simulink model "EX001_FCHEV"  (R2020b)
settings: Solver=ode23tb  StartTime=0.0  StopTime=20e3  MaxStep=1  RelTol=1e-4
libraries: component_lib x75, pid_lib x3, simulink x2, base_lib x1
settings Model: Creator=maxjo65  LastModifiedBy=CJ

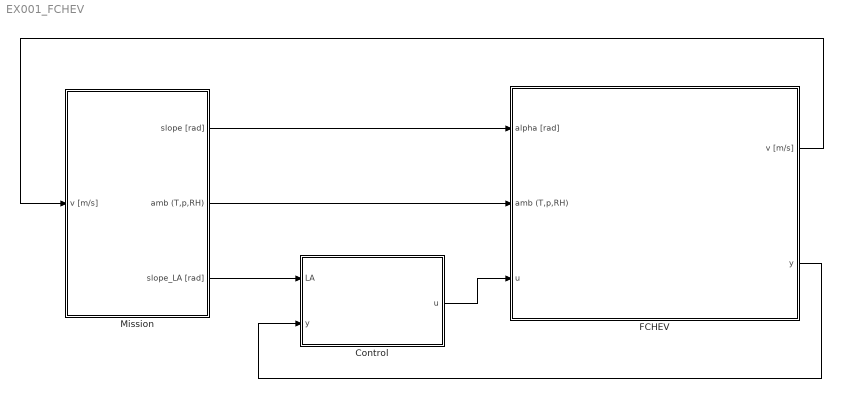
== system EX001_FCHEV ==
  Control : Subsystem
  FCHEV : Subsystem
  Mission : Subsystem
  wires:
  FCHEV/1(v [m/s]) -> Mission/1(v [m/s])
  Mission/1(slope [rad]) -> FCHEV/1(alpha [rad])
  Mission/2(amb (T,p,RH)) -> FCHEV/2(amb (T,p,RH))
  Mission/3(slope_LA [rad]) -> Control/1(LA)
  Control/1(u) -> FCHEV/3(u)
  FCHEV/2(y) -> Control/2(y)

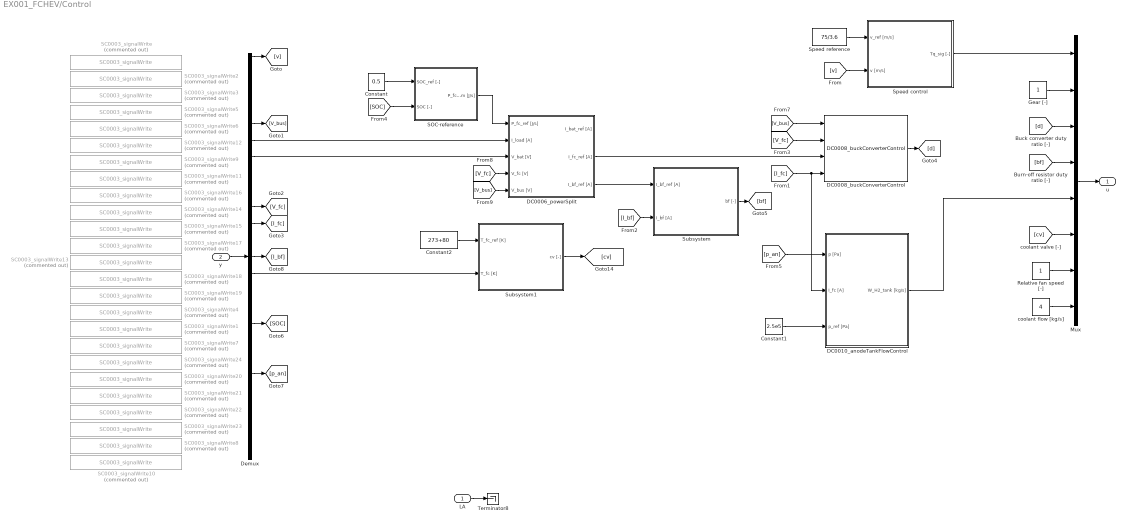
== system EX001_FCHEV/Control ==
  LA : Inport
  y : Inport  Port=2
  Constant : Constant  Value=0.5
  Constant1 : Constant  Value=2.5e5
  Constant2 : Constant  Value=273+80
  DC0006_powerSplit : Subsystem  mask{P_fc_max=400e3, P_fc_min=10e3, T_s=1, I_bt_max=600, I_bt_min=-300}
      mask prompts: P_fc_max "Max. FC power [J/s]:"; P_fc_min "Min. FC power [J/s]:"; T_s "FC Dynamic load time constant [s]:"; I_bt_max "Max. battery current [A]:"; I_bt_min "Min. battery current [A]:"
  DC0008_buckConverterControl : component_lib/Data & Control/DC0008_buckConverterControl  SystemSampleTime=-1  VariantActivationTime=update diagram  Latency=0  AutoFrameSizeCalculation=off
  DC0010_anodeTankFlowControl : Subsystem  mask{n_cell=450*2}
      mask prompts: n_cell "Nr. of cells [-]"
  Demux : Demux  Outputs=25
  Gear [-] : Constant
  Mux : Mux  Inputs=8
  Relative fan speed [-] : Constant
  SC0003_signalWrite : component_lib/Data & Control/SC0003_signalWrite  Commented=on  SigName=velocity
  SC0003_signalWrite1 : component_lib/Data & Control/SC0003_signalWrite  Commented=on  SigName=stateOfCharge
  SC0003_signalWrite10 : component_lib/Data & Control/SC0003_signalWrite  Commented=on  SigName=empty
  SC0003_signalWrite11 : component_lib/Data & Control/SC0003_signalWrite  Commented=on  SigName=batteryCurrent
  SC0003_signalWrite12 : component_lib/Data & Control/SC0003_signalWrite  Commented=on  SigName=loadCurrent
  SC0003_signalWrite13 : component_lib/Data & Control/SC0003_signalWrite  Commented=on  SigName=burnOffCurrent
  SC0003_signalWrite14 : component_lib/Data & Control/SC0003_signalWrite  Commented=on  SigName=fuelCellVoltage
  SC0003_signalWrite15 : component_lib/Data & Control/SC0003_signalWrite  Commented=on  SigName=fuelCellCurrent
  SC0003_signalWrite16 : component_lib/Data & Control/SC0003_signalWrite  Commented=on  SigName=batteryPower
  SC0003_signalWrite17 : component_lib/Data & Control/SC0003_signalWrite  Commented=on  SigName=fuelCellPower
  SC0003_signalWrite18 : component_lib/Data & Control/SC0003_signalWrite  Commented=on  SigName=fuelCellTemperature
  SC0003_signalWrite19 : component_lib/Data & Control/SC0003_signalWrite  Commented=on  SigName=motorTemperature
  SC0003_signalWrite2 : component_lib/Data & Control/SC0003_signalWrite  Commented=on  SigName=motorTorque
  SC0003_signalWrite20 : component_lib/Data & Control/SC0003_signalWrite  Commented=on  SigName=anodeSupplyPressure
  SC0003_signalWrite21 : component_lib/Data & Control/SC0003_signalWrite  Commented=on  SigName=anodeSupplyHumidity
  SC0003_signalWrite22 : component_lib/Data & Control/SC0003_signalWrite  Commented=on  SigName=cathodePressure
  SC0003_signalWrite23 : component_lib/Data & Control/SC0003_signalWrite  Commented=on  SigName=cathodeHumidity
  SC0003_signalWrite24 : component_lib/Data & Control/SC0003_signalWrite  Commented=on  SigName=anodePrimaryFlow
  SC0003_signalWrite3 : component_lib/Data & Control/SC0003_signalWrite  Commented=on  SigName=maxMotorTorque
  SC0003_signalWrite4 : component_lib/Data & Control/SC0003_signalWrite  Commented=on  SigName=powerElectronicsTemperature
  SC0003_signalWrite5 : component_lib/Data & Control/SC0003_signalWrite  Commented=on  SigName=motorSpeed
  SC0003_signalWrite6 : component_lib/Data & Control/SC0003_signalWrite  Commented=on  SigName=busVoltage
  SC0003_signalWrite7 : component_lib/Data & Control/SC0003_signalWrite  Commented=on  SigName=anodePrimaryPressure
  SC0003_signalWrite8 : component_lib/Data & Control/SC0003_signalWrite  Commented=on  SigName=anodePrimaryPressure
  SC0003_signalWrite9 : component_lib/Data & Control/SC0003_signalWrite  Commented=on  SigName=batteryVoltage
  SOC-reference : Subsystem
  Speed control : Subsystem
  Speed reference : Constant  Value=75/3.6
  Subsystem : Subsystem
  Subsystem1 : Subsystem
  Terminator8 : Terminator
  coolant flow [kg/s] : Constant  Value=4
  u : Outport
  wires:
  y/1 -> Demux/1
  Demux/1 -> [v]
  Mux/1 -> u/1
  Speed reference/1 -> Speed control/1(v_ref [m/s])
  Speed control/1(Tq_sig [-]) -> Mux/1
  [v] -> Speed control/2(v [m/s])
  Gear [-]/1 -> Mux/2
  [V_bus] -> DC0008_buckConverterControl/1
  [V_fc] -> DC0008_buckConverterControl/2
  DC0006_powerSplit/2(I_fc_ref [A]) -> DC0008_buckConverterControl/3
  DC0006_powerSplit/3(I_bf_ref [A]) -> Subsystem/1(I_bf_ref [A])
  Demux/6 -> DC0006_powerSplit/2(I_load [A])
  Demux/7 -> DC0006_powerSplit/3(V_bat [V])
  Demux/5 -> [V_bus]
  Demux/10 -> [V_fc]
  Demux/11 -> [I_fc]
  DC0008_buckConverterControl/1 -> [d]
  [d] -> Mux/3
  [bf] -> Mux/4
  Subsystem/1(bf [-]) -> [bf]
  [cv] -> Mux/6
  [I_fc] -> DC0010_anodeTankFlowControl/2(I_fc [A]), DC0008_buckConverterControl/4
  [I_bf] -> Subsystem/2(I_bf [A])
  Constant2/1 -> Subsystem1/1(T_fc_ref [K])
  Subsystem1/1(cv [-]) -> [cv]
  Demux/13 -> [I_bf]
  Demux/14 -> Subsystem1/2(T_fc [K])
  Relative fan speed [-]/1 -> Mux/7
  coolant flow [kg/s]/1 -> Mux/8
  LA/1 -> Terminator8/1
  [V_fc] -> DC0006_powerSplit/4(V_fc [V])
  [V_bus] -> DC0006_powerSplit/5(V_bus [V])
  Demux/17 -> [SOC]
  SOC-reference/1(P_fc_nom [J/s]) -> DC0006_powerSplit/1(P_fc_ref [J/s])
  Constant/1 -> SOC-reference/1(SOC_ref [-])
  [SOC] -> SOC-reference/2(SOC [-])
  DC0010_anodeTankFlowControl/1(W_H2_tank [kg/s]) -> Mux/5
  Demux/20 -> [p_an]
  [p_an] -> DC0010_anodeTankFlowControl/1(p [Pa])
  Constant1/1 -> DC0010_anodeTankFlowControl/3(p_ref [Pa])

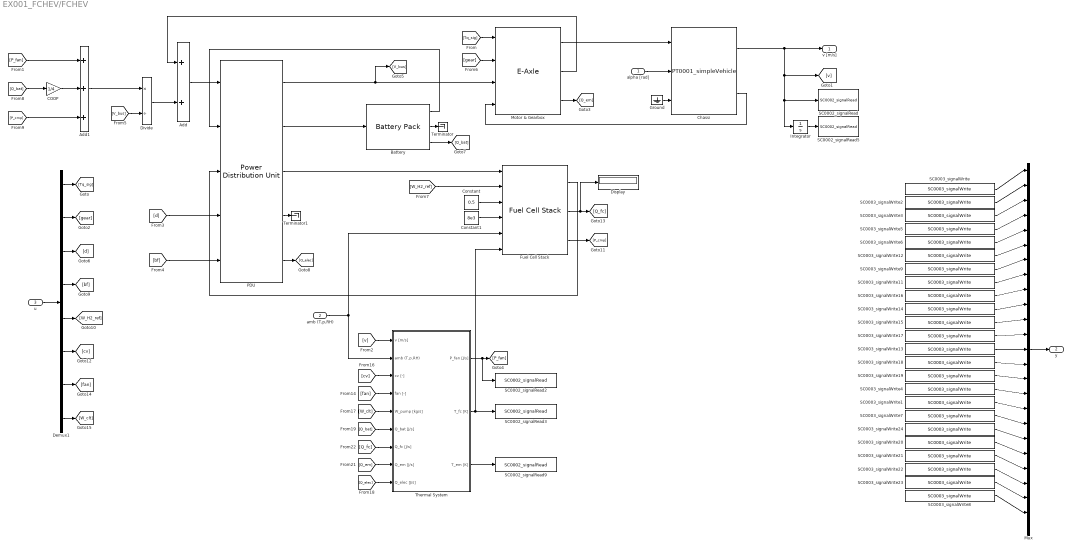
== system EX001_FCHEV/FCHEV ==
  alpha [rad] : Inport
  amb (T,p,RH) : Inport  Port=2
  u : Inport  Port=3
  Add : Sum
  Add1 : Sum  Inputs=3
  Battery : component_lib/Battery Pack  SOC_0=0.5  Nx=80  Ny=100  T_bat=273 + 20
  COOP : Gain  Gain=1/4
  Chassi : component_lib/Powertrain/PT0001_simpleVehicle  m=40e3  r_w=0.5  A_f=10  C_d=0.5  rho_air=1.225  c_r0=0.0060  c_r1=2.3e-7  gain=600  v0=75/3.6  x0=0
  Constant : Constant  Value=0.5
  Constant1 : Constant  Value=8e3
  Demux1 : Demux  Outputs=8
  Display : Display
  Divide : Product  Inputs=*/
  Fuel Cell Stack : component_lib/Fuel Cell Stack  n=450*2
  Ground : Ground
  Integrator : Integrator
  Motor & Gearbox : component_lib/E-Axle  n=3
  Mux : Mux  Inputs=25
  PDU : component_lib/Power Distribution Unit  R_bf=0.5
  SC0002_signalRead : component_lib/Data & Control/SC0002_signalRead  SigName=velocity
  SC0002_signalRead2 : component_lib/Data & Control/SC0002_signalRead  SigName=fanPower
  SC0002_signalRead3 : component_lib/Data & Control/SC0002_signalRead  SigName=fuelCellTemperature
  SC0002_signalRead5 : component_lib/Data & Control/SC0002_signalRead  SigName=distance
  SC0002_signalRead9 : component_lib/Data & Control/SC0002_signalRead  SigName=motorTemperature
  SC0003_signalWrite : component_lib/Data & Control/SC0003_signalWrite  SigName=velocity
  SC0003_signalWrite1 : component_lib/Data & Control/SC0003_signalWrite  SigName=stateOfCharge
  SC0003_signalWrite11 : component_lib/Data & Control/SC0003_signalWrite  SigName=batteryCurrent
  SC0003_signalWrite12 : component_lib/Data & Control/SC0003_signalWrite  SigName=loadCurrent
  SC0003_signalWrite13 : component_lib/Data & Control/SC0003_signalWrite  SigName=burnOffCurrent
  SC0003_signalWrite14 : component_lib/Data & Control/SC0003_signalWrite  SigName=fuelCellVoltage
  SC0003_signalWrite15 : component_lib/Data & Control/SC0003_signalWrite  SigName=fuelCellCurrent
  SC0003_signalWrite16 : component_lib/Data & Control/SC0003_signalWrite  SigName=batteryPower
  SC0003_signalWrite17 : component_lib/Data & Control/SC0003_signalWrite  SigName=fuelCellPower
  SC0003_signalWrite18 : component_lib/Data & Control/SC0003_signalWrite  SigName=fuelCellTemperature
  SC0003_signalWrite19 : component_lib/Data & Control/SC0003_signalWrite  SigName=motorTemperature
  SC0003_signalWrite2 : component_lib/Data & Control/SC0003_signalWrite  SigName=motorTorque
  SC0003_signalWrite20 : component_lib/Data & Control/SC0003_signalWrite  SigName=anodeSupplyPressure
  SC0003_signalWrite21 : component_lib/Data & Control/SC0003_signalWrite  SigName=anodeSupplyHumidity
  SC0003_signalWrite22 : component_lib/Data & Control/SC0003_signalWrite  SigName=cathodePressure
  SC0003_signalWrite23 : component_lib/Data & Control/SC0003_signalWrite  SigName=cathodeHumidity
  SC0003_signalWrite24 : component_lib/Data & Control/SC0003_signalWrite  SigName=anodePrimaryFlow
  SC0003_signalWrite3 : component_lib/Data & Control/SC0003_signalWrite  SigName=maxMotorTorque
  SC0003_signalWrite4 : component_lib/Data & Control/SC0003_signalWrite  SigName=powerElectronicsTemperature
  SC0003_signalWrite5 : component_lib/Data & Control/SC0003_signalWrite  SigName=motorSpeed
  SC0003_signalWrite6 : component_lib/Data & Control/SC0003_signalWrite  SigName=busVoltage
  SC0003_signalWrite7 : component_lib/Data & Control/SC0003_signalWrite  SigName=anodePrimaryPressure
  SC0003_signalWrite8 : component_lib/Data & Control/SC0003_signalWrite  SigName=anodePrimaryPressure
  SC0003_signalWrite9 : component_lib/Data & Control/SC0003_signalWrite  SigName=batteryVoltage
  Terminator : Terminator
  Terminator1 : Terminator
  Thermal System : Subsystem
  v [m/s] : Outport
  y : Outport  Port=2
  wires:
  Battery/1 -> PDU/2
  Fuel Cell Stack/1 -> PDU/3
  PDU/2 -> Battery/1
  PDU/3 -> Fuel Cell Stack/1
  Motor & Gearbox/3 -> [Q_em]
  Motor & Gearbox/1 -> Chassi/1
  Chassi/1 -> v [m/s]/1, [v], SC0002_signalRead/1, Integrator/1
  Chassi/2 -> Motor & Gearbox/4
  Motor & Gearbox/2 -> Add/1
  PDU/5 -> [Q_elec]
  Battery/3 -> [Q_bat]
  PDU/1 -> [V_bus], Motor & Gearbox/3
  alpha [rad]/1 -> Chassi/2
  u/1 -> Demux1/1
  Demux1/2 -> [gear]
  Demux1/1 -> [Tq_sig]
  [Tq_sig] -> Motor & Gearbox/1
  [gear] -> Motor & Gearbox/2
  Demux1/3 -> [d]
  Demux1/4 -> [bf]
  [d] -> PDU/4
  [bf] -> PDU/5
  Demux1/6 -> [cv]
  Mux/1 -> y/1
  Thermal System/2(T_fc [K]) -> Fuel Cell Stack/6, SC0002_signalRead3/1
  Demux1/7 -> [fan]
  Demux1/8 -> [W_clt]
  amb (T,p,RH)/1 -> Fuel Cell Stack/5, Thermal System/2(amb (T,p,RH))
  Thermal System/3(T_em [K]) -> SC0002_signalRead9/1
  [v] -> Thermal System/1(v [m/s])
  [fan] -> Thermal System/4(fan [-])
  [W_clt] -> Thermal System/5(W_pump [kg/s])
  [cv] -> Thermal System/3(cv [-])
  [Q_elec] -> Thermal System/9(Q_elec [J/s])
  [Q_bat] -> Thermal System/6(Q_bat [J/s])
  [Q_em] -> Thermal System/8(Q_em [J/s])
  [Q_fc] -> Thermal System/7(Q_fc [J/s])
  SC0003_signalWrite4/1 -> Mux/16
  SC0003_signalWrite2/1 -> Mux/2
  SC0003_signalWrite19/1 -> Mux/15
  SC0003_signalWrite/1 -> Mux/1
  SC0003_signalWrite17/1 -> Mux/12
  SC0003_signalWrite16/1 -> Mux/9
  SC0003_signalWrite13/1 -> Mux/13
  SC0003_signalWrite6/1 -> Mux/5
  SC0003_signalWrite15/1 -> Mux/11
  SC0003_signalWrite5/1 -> Mux/4
  SC0003_signalWrite9/1 -> Mux/7
  SC0003_signalWrite3/1 -> Mux/3
  SC0003_signalWrite11/1 -> Mux/8
  SC0003_signalWrite12/1 -> Mux/6
  SC0003_signalWrite18/1 -> Mux/14
  SC0003_signalWrite14/1 -> Mux/10
  Integrator/1 -> SC0002_signalRead5/1
  Ground/1 -> Chassi/3
  SC0003_signalWrite1/1 -> Mux/17
  Add/1 -> PDU/1
  Battery/2 -> Terminator/1
  Thermal System/1(P_fan [J/s]) -> SC0002_signalRead2/1, [P_fan]
  [Q_bat] -> COOP/1
  [P_fan] -> Add1/1
  COOP/1 -> Add1/2
  Add1/1 -> Divide/1
  Divide/1 -> Add/2
  [V_bus] -> Divide/2
  [P_cmp] -> Add1/3
  PDU/4 -> Terminator1/1
  Fuel Cell Stack/2 -> Display/1, [Q_fc]
  Fuel Cell Stack/3 -> [P_cmp]
  Constant/1 -> Fuel Cell Stack/3
  Constant1/1 -> Fuel Cell Stack/4
  Demux1/5 -> [W_H2_ref]
  [W_H2_ref] -> Fuel Cell Stack/2
  SC0003_signalWrite7/1 -> Mux/18
  SC0003_signalWrite22/1 -> Mux/22
  SC0003_signalWrite23/1 -> Mux/23
  SC0003_signalWrite21/1 -> Mux/21
  SC0003_signalWrite20/1 -> Mux/20
  SC0003_signalWrite24/1 -> Mux/19
  SC0003_signalWrite8/1 -> Mux/24

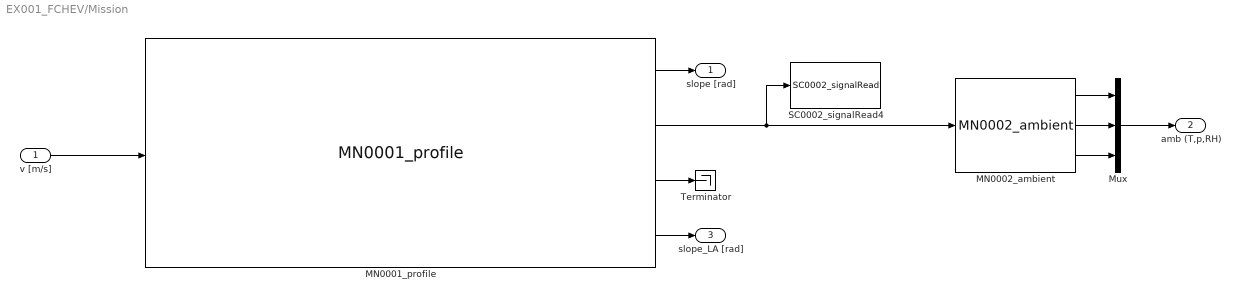
== system EX001_FCHEV/Mission ==
  v [m/s] : Inport
  MN0001_profile : component_lib/Mission/MN0001_profile  profile=KoblenzTrier.mat  x0=0  N_lookahead=100
  MN0002_ambient : component_lib/Mission/MN0002_ambient  p_0=1.01e5  T_0=273 + 45  RH_0=0.2
  Mux : Mux  Inputs=3
  SC0002_signalRead4 : component_lib/Data & Control/SC0002_signalRead  SigName=altitude
  Terminator : Terminator
  slope [rad] : Outport
  amb (T,p,RH) : Outport  Port=2
  slope_LA [rad] : Outport  Port=3
  wires:
  Mux/1 -> amb (T,p,RH)/1
  MN0001_profile/2 -> MN0002_ambient/1, SC0002_signalRead4/1
  MN0001_profile/1 -> slope [rad]/1
  MN0002_ambient/3 -> Mux/3
  MN0002_ambient/1 -> Mux/1
  MN0002_ambient/2 -> Mux/2
  v [m/s]/1 -> MN0001_profile/1
  MN0001_profile/4 -> slope_LA [rad]/1
  MN0001_profile/3 -> Terminator/1

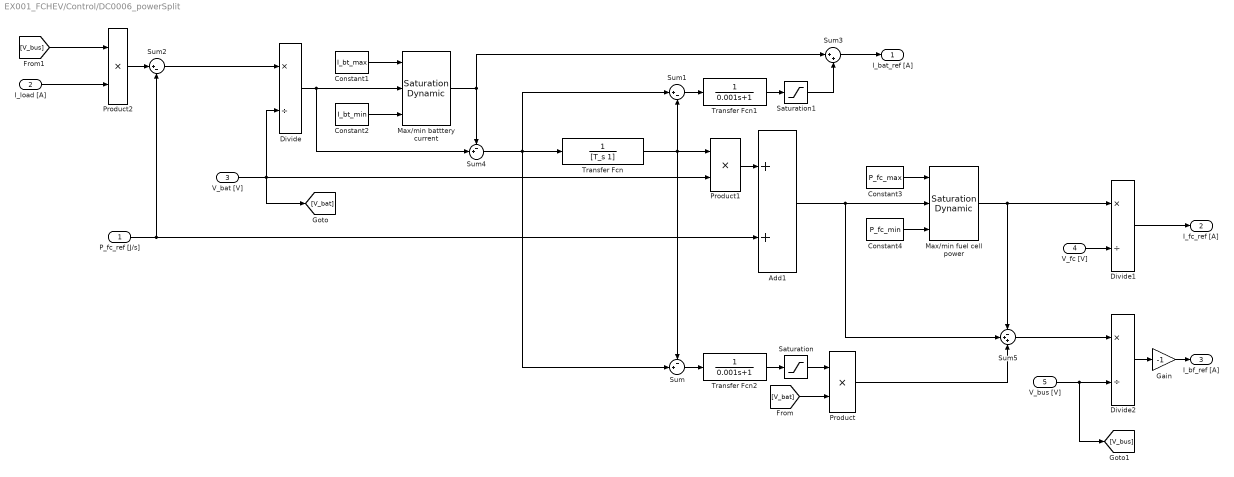
== system EX001_FCHEV/Control/DC0006_powerSplit ==
  P_fc_ref [J/s] : Inport
  I_load [A] : Inport  Port=2
  V_bat [V] : Inport  Port=3
  V_fc [V] : Inport  Port=4
  V_bus [V] : Inport  Port=5
  Add1 : Sum
  Constant1 : Constant  Value=I_bt_max
  Constant2 : Constant  Value=I_bt_min
  Constant3 : Constant  Value=P_fc_max
  Constant4 : Constant  Value=P_fc_min
  Divide : Product  Inputs=*/
  Divide1 : Product  Inputs=*/
  Divide2 : Product  Inputs=*/
  Gain : Gain  Gain=-1
  Max/min batttery current : simulink/Discontinuities/Saturation Dynamic  OutMin=[]  OutMax=[]  OutDataTypeStr=Inherit: Same as second input  OutDataType=fixdt(1, 16)  OutScaling=2^-10  DoSatur=off
  Max/min fuel cell power : simulink/Discontinuities/Saturation Dynamic  OutMin=[]  OutMax=[]  OutDataTypeStr=Inherit: Same as second input  OutDataType=fixdt(1, 16)  OutScaling=2^-10  DoSatur=off
  Product : Product
  Product1 : Product
  Product2 : Product
  Saturation : Saturate  UpperLimit=0  LowerLimit=-inf
  Saturation1 : Saturate  UpperLimit=inf  LowerLimit=0
  Sum : Sum  Inputs=-+|
  Sum1 : Sum  Inputs=|+-
  Sum2 : Sum  Inputs=|+-
  Sum3 : Sum  Inputs=|++
  Sum4 : Sum  Inputs=-+|
  Sum5 : Sum  Inputs=-++
  Transfer Fcn : TransferFcn  Denominator=[T_s 1]
  Transfer Fcn1 : TransferFcn  Denominator=[0.001 1]
  Transfer Fcn2 : TransferFcn  Denominator=[0.001 1]
  I_bat_ref [A] : Outport
  I_fc_ref [A] : Outport  Port=2
  I_bf_ref [A] : Outport  Port=3
  wires:
  Gain/1 -> I_bf_ref [A]/1
  [V_bus] -> Product2/1
  I_load [A]/1 -> Product2/2
  Product2/1 -> Sum2/1
  Transfer Fcn2/1 -> Saturation/1
  Sum/1 -> Transfer Fcn2/1
  Transfer Fcn1/1 -> Saturation1/1
  Sum1/1 -> Transfer Fcn1/1
  Sum3/1 -> I_bat_ref [A]/1
  Saturation1/1 -> Sum3/2
  Product/1 -> Sum5/3
  Saturation/1 -> Product/1
  [V_bat] -> Product/2
  Transfer Fcn/1 -> Sum/1, Product1/1, Sum1/2
  Sum4/1 -> Transfer Fcn/1, Sum/2, Sum1/1
  Max/min batttery current/1 -> Sum4/1, Sum3/1
  Product1/1 -> Add1/1
  V_fc [V]/1 -> Divide1/2
  Divide2/1 -> Gain/1
  V_bus [V]/1 -> Divide2/2, [V_bus]
  Sum5/1 -> Divide2/1
  Max/min fuel cell power/1 -> Divide1/1, Sum5/1
  Constant4/1 -> Max/min fuel cell power/3
  Constant3/1 -> Max/min fuel cell power/1
  Add1/1 -> Max/min fuel cell power/2, Sum5/2
  Constant2/1 -> Max/min batttery current/3
  Constant1/1 -> Max/min batttery current/1
  Divide/1 -> Sum4/2, Max/min batttery current/2
  P_fc_ref [J/s]/1 -> Add1/2, Sum2/2
  V_bat [V]/1 -> Divide/2, [V_bat], Product1/2
  Divide1/1 -> I_fc_ref [A]/1
  Sum2/1 -> Divide/1

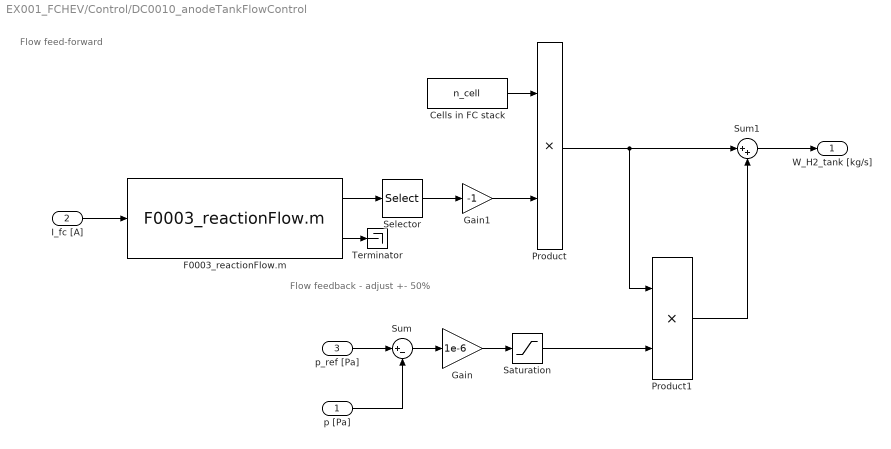
== system EX001_FCHEV/Control/DC0010_anodeTankFlowControl ==
  note: Flow feed-forward
  note: Flow feedback - adjust +- 50%
  p [Pa] : Inport
  I_fc [A] : Inport  Port=2
  p_ref [Pa] : Inport  Port=3
  Cells in FC stack : Constant  Value=n_cell
  F0003_reactionFlow.m : base_lib/F0003_pukrushpan2004/F0003_reactionFlow.m  SystemSampleTime=-1  VariantActivationTime=update diagram  Latency=0  AutoFrameSizeCalculation=off
  Gain : Gain  Gain=1e-6
  Gain1 : Gain  Gain=-1
  Product : Product
  Product1 : Product
  Saturation : Saturate
  Selector : Selector  InputPortWidth=4  IndexOptions=Index vector (dialog)  Indices=1  OutputSizes=1
  Sum : Sum  Inputs=|+-
  Sum1 : Sum  Inputs=|++
  Terminator : Terminator
  W_H2_tank [kg/s] : Outport
  wires:
  Saturation/1 -> Product1/2
  Gain/1 -> Saturation/1
  Product1/1 -> Sum1/2
  Sum/1 -> Gain/1
  Sum1/1 -> W_H2_tank [kg/s]/1
  Product/1 -> Product1/1, Sum1/1
  p [Pa]/1 -> Sum/2
  p_ref [Pa]/1 -> Sum/1
  Cells in FC stack/1 -> Product/1
  F0003_reactionFlow.m/2 -> Terminator/1
  I_fc [A]/1 -> F0003_reactionFlow.m/1
  F0003_reactionFlow.m/1 -> Selector/1
  Selector/1 -> Gain1/1
  Gain1/1 -> Product/2

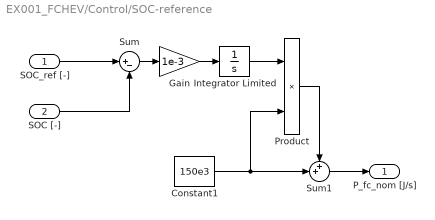
== system EX001_FCHEV/Control/SOC-reference ==
  SOC_ref [-] : Inport
  SOC [-] : Inport  Port=2
  Constant1 : Constant  Value=150e3
  Gain : Gain  Gain=1e-3
  Integrator Limited : Integrator  LimitOutput=on  UpperSaturationLimit=0.3  LowerSaturationLimit=-0.3
  Product : Product
  Sum : Sum  Inputs=|+-
  Sum1 : Sum  Inputs=++|
  P_fc_nom [J/s] : Outport
  wires:
  Product/1 -> Sum1/1
  Integrator Limited/1 -> Product/1
  Sum1/1 -> P_fc_nom [J/s]/1
  Constant1/1 -> Sum1/2, Product/2
  Sum/1 -> Gain/1
  SOC [-]/1 -> Sum/2
  Gain/1 -> Integrator Limited/1
  SOC_ref [-]/1 -> Sum/1

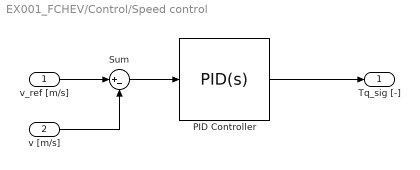
== system EX001_FCHEV/Control/Speed control ==
  v_ref [m/s] : Inport
  v [m/s] : Inport  Port=2
  PID Controller : pid_lib/PID Controller  Controller=PID  Form=Parallel  TimeDomain=Continuous-time  UseExternalTs=off  SampleTime=-1  IntegratorMethod=Forward Euler  FilterMethod=Forward Euler  ControllerParametersSource=internal  P=10  I=1e-1  D=0  UseFilter=on  N=100  TunerSelectOption=Transfer Function Based (PID Tuner App)  ZeroCross=off  InitialConditionSource=internal  InitialConditionForIntegrator=0  InitialConditionForFilter=0  DifferentiatorICPrevScaledInput=0  ExternalReset=none  TrackingMode=off  Kt=1  LimitOutput=on  SatLimitsSource=internal  UpperSaturationLimit=1  LowerSaturationLimit=-1  LinearizeAsGain=on  AntiWindupMode=clamping  Kb=1  POutMin=[]  POutMax=[]  IOutMin=[]  IOutMax=[]  DOutMin=[]  DOutMax=[]  NOutMin=[]  NOutMax=[]  SumOutMin=[]  SumOutMax=[]  SaturationOutMin=[]  SaturationOutMax=[]  PParamMin=[]  PParamMax=[]  IParamMin=[]  IParamMax=[]  DParamMin=[]  DParamMax=[]  NParamMin=[]  NParamMax=[]  KbParamMin=[]  KbParamMax=[]  KtParamMin=[]  KtParamMax=[]  KbOutMin=[]  KbOutMax=[]  KtOutMin=[]  KtOutMax=[]  IntegratorOutMin=[]  IntegratorOutMax=[]  FilterOutMin=[]  FilterOutMax=[]  SumI1OutMin=[]  SumI1OutMax=[]  SumI2OutMin=[]  SumI2OutMax=[]  SumI3OutMin=[]  SumI3OutMax=[]  SumI4OutMin=[]  SumI4OutMax=[]  SumDOutMin=[]  SumDOutMax=[]  DifferentiatorOutMin=[]  DifferentiatorOutMax=[]  FilterDiffOutCoefMin=[]  FilterDiffOutCoefMax=[]  ReciprocalOutMin=[]  ReciprocalOutMax=[]  SumDenOutMin=[]  SumDenOutMax=[]  SumNumOutMin=[]  SumNumOutMax=[]  DivideOutMin=[]  DivideOutMax=[]  UdiffTsProdOutMin=[]  UdiffTsProdOutMax=[]  NTsProdOutMin=[]  NTsProdOutMax=[]  UintegralTsProdOutMin=[]  UintegralTsProdOutMax=[]  UngainTsProdOutMin=[]  UngainTsProdOutMax=[]  IntegratorContinuousStateAttributes=''  IntegratorStateMustResolveToSignalObject=off  IntegratorRTWStateStorageClass=Auto  FilterContinuousStateAttributes=''  FilterStateMustResolveToSignalObject=off  FilterRTWStateStorageClass=Auto  ParallelPVariant=InternalParameters  IdealPVariant=Disabled  IVariant=InternalParameters  DVariant=InternalParameters  IntegratorVariant=Continuous  SatVariant=Enabled  AWVariant=ContClampingParallel  PCopyVariant=Disabled  TRVariant=Disabled  FdbkBlocksVariant=Forward  IdealPFdbkVariant=Disabled  SatFdbkVariant=Disabled  DerivativeFilterVariant=ContFilter  NVariant=InternalParameters  NCopyVariant=Disabled  FilterICVariant=InternalICsFilter  IntegratorICVariant=InternalICs  ExternalResetVariant=Disabled  TRSumVariant=Passthrough  SumFdbkVariant=Disabled  SumVariant=Sum_PID  TsampFilterVariant=InternalTs  TsampNgainVariant=Passthrough  TsampIntegralVariant=Passthrough  ExternalSaturationOutDataTypeStr=Inherit: Same as second input
  Sum : Sum  Inputs=|+-
  Tq_sig [-] : Outport
  wires:
  PID Controller/1 -> Tq_sig [-]/1
  Sum/1 -> PID Controller/1
  v_ref [m/s]/1 -> Sum/1
  v [m/s]/1 -> Sum/2

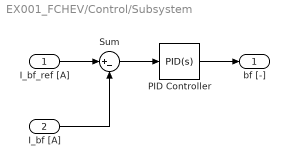
== system EX001_FCHEV/Control/Subsystem ==
  I_bf_ref [A] : Inport
  I_bf [A] : Inport  Port=2
  PID Controller : pid_lib/PID Controller  Controller=PID  Form=Parallel  TimeDomain=Continuous-time  UseExternalTs=off  SampleTime=-1  IntegratorMethod=Forward Euler  FilterMethod=Forward Euler  ControllerParametersSource=internal  P=1e-3  I=1e-3  D=0  UseFilter=on  N=100  TunerSelectOption=Transfer Function Based (PID Tuner App)  InitialConditionSource=internal  InitialConditionForIntegrator=0  InitialConditionForFilter=0  DifferentiatorICPrevScaledInput=0  ExternalReset=none  TrackingMode=off  Kt=1  LimitOutput=off  SatLimitsSource=internal  UpperSaturationLimit=inf  LowerSaturationLimit=-inf  LinearizeAsGain=on  AntiWindupMode=none  Kb=1  POutMin=[]  POutMax=[]  IOutMin=[]  IOutMax=[]  DOutMin=[]  DOutMax=[]  NOutMin=[]  NOutMax=[]  SumOutMin=[]  SumOutMax=[]  SaturationOutMin=[]  SaturationOutMax=[]  PParamMin=[]  PParamMax=[]  IParamMin=[]  IParamMax=[]  DParamMin=[]  DParamMax=[]  NParamMin=[]  NParamMax=[]  KbParamMin=[]  KbParamMax=[]  KtParamMin=[]  KtParamMax=[]  KbOutMin=[]  KbOutMax=[]  KtOutMin=[]  KtOutMax=[]  IntegratorOutMin=[]  IntegratorOutMax=[]  FilterOutMin=[]  FilterOutMax=[]  SumI1OutMin=[]  SumI1OutMax=[]  SumI2OutMin=[]  SumI2OutMax=[]  SumI3OutMin=[]  SumI3OutMax=[]  SumI4OutMin=[]  SumI4OutMax=[]  SumDOutMin=[]  SumDOutMax=[]  DifferentiatorOutMin=[]  DifferentiatorOutMax=[]  FilterDiffOutCoefMin=[]  FilterDiffOutCoefMax=[]  ReciprocalOutMin=[]  ReciprocalOutMax=[]  SumDenOutMin=[]  SumDenOutMax=[]  SumNumOutMin=[]  SumNumOutMax=[]  DivideOutMin=[]  DivideOutMax=[]  UdiffTsProdOutMin=[]  UdiffTsProdOutMax=[]  NTsProdOutMin=[]  NTsProdOutMax=[]  UintegralTsProdOutMin=[]  UintegralTsProdOutMax=[]  UngainTsProdOutMin=[]  UngainTsProdOutMax=[]  IntegratorContinuousStateAttributes=''  IntegratorStateMustResolveToSignalObject=off  IntegratorRTWStateStorageClass=Auto  FilterContinuousStateAttributes=''  FilterStateMustResolveToSignalObject=off  FilterRTWStateStorageClass=Auto  ParallelPVariant=InternalParameters  IdealPVariant=Disabled  IVariant=InternalParameters  DVariant=InternalParameters  IntegratorVariant=Continuous  SatVariant=Disabled  AWVariant=Passthrough  PCopyVariant=Disabled  TRVariant=Disabled  FdbkBlocksVariant=Forward  IdealPFdbkVariant=Disabled  SatFdbkVariant=Disabled  DerivativeFilterVariant=ContFilter  NVariant=InternalParameters  NCopyVariant=Disabled  FilterICVariant=InternalICsFilter  IntegratorICVariant=InternalICs  ExternalResetVariant=Disabled  TRSumVariant=Passthrough  SumFdbkVariant=Disabled  SumVariant=Sum_PID  TsampFilterVariant=InternalTs  TsampNgainVariant=Passthrough  TsampIntegralVariant=Passthrough  ExternalSaturationOutDataTypeStr=Inherit: Same as second input
  Sum : Sum  Inputs=|+-
  bf [-] : Outport
  wires:
  I_bf_ref [A]/1 -> Sum/1
  Sum/1 -> PID Controller/1
  PID Controller/1 -> bf [-]/1
  I_bf [A]/1 -> Sum/2

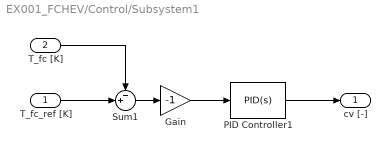
== system EX001_FCHEV/Control/Subsystem1 ==
  T_fc_ref [K] : Inport
  T_fc [K] : Inport  Port=2
  Gain : Gain  Gain=-1
  PID Controller1 : pid_lib/PID Controller  Controller=PID  Form=Parallel  TimeDomain=Continuous-time  UseExternalTs=off  SampleTime=-1  IntegratorMethod=Forward Euler  FilterMethod=Forward Euler  ControllerParametersSource=internal  P=1e-2  I=1e-2  D=0  UseFilter=on  N=100  TunerSelectOption=Transfer Function Based (PID Tuner App)  ZeroCross=off  InitialConditionSource=internal  InitialConditionForIntegrator=0.5  InitialConditionForFilter=0  DifferentiatorICPrevScaledInput=0  ExternalReset=none  TrackingMode=off  Kt=1  LimitOutput=on  SatLimitsSource=internal  UpperSaturationLimit=0.95  LowerSaturationLimit=0.05  LinearizeAsGain=on  AntiWindupMode=clamping  Kb=1  POutMin=[]  POutMax=[]  IOutMin=[]  IOutMax=[]  DOutMin=[]  DOutMax=[]  NOutMin=[]  NOutMax=[]  SumOutMin=[]  SumOutMax=[]  SaturationOutMin=[]  SaturationOutMax=[]  PParamMin=[]  PParamMax=[]  IParamMin=[]  IParamMax=[]  DParamMin=[]  DParamMax=[]  NParamMin=[]  NParamMax=[]  KbParamMin=[]  KbParamMax=[]  KtParamMin=[]  KtParamMax=[]  KbOutMin=[]  KbOutMax=[]  KtOutMin=[]  KtOutMax=[]  IntegratorOutMin=[]  IntegratorOutMax=[]  FilterOutMin=[]  FilterOutMax=[]  SumI1OutMin=[]  SumI1OutMax=[]  SumI2OutMin=[]  SumI2OutMax=[]  SumI3OutMin=[]  SumI3OutMax=[]  SumI4OutMin=[]  SumI4OutMax=[]  SumDOutMin=[]  SumDOutMax=[]  DifferentiatorOutMin=[]  DifferentiatorOutMax=[]  FilterDiffOutCoefMin=[]  FilterDiffOutCoefMax=[]  ReciprocalOutMin=[]  ReciprocalOutMax=[]  SumDenOutMin=[]  SumDenOutMax=[]  SumNumOutMin=[]  SumNumOutMax=[]  DivideOutMin=[]  DivideOutMax=[]  UdiffTsProdOutMin=[]  UdiffTsProdOutMax=[]  NTsProdOutMin=[]  NTsProdOutMax=[]  UintegralTsProdOutMin=[]  UintegralTsProdOutMax=[]  UngainTsProdOutMin=[]  UngainTsProdOutMax=[]  IntegratorContinuousStateAttributes=''  IntegratorStateMustResolveToSignalObject=off  IntegratorRTWStateStorageClass=Auto  FilterContinuousStateAttributes=''  FilterStateMustResolveToSignalObject=off  FilterRTWStateStorageClass=Auto  ParallelPVariant=InternalParameters  IdealPVariant=Disabled  IVariant=InternalParameters  DVariant=InternalParameters  IntegratorVariant=Continuous  SatVariant=Enabled  AWVariant=ContClampingParallel  PCopyVariant=Disabled  TRVariant=Disabled  FdbkBlocksVariant=Forward  IdealPFdbkVariant=Disabled  SatFdbkVariant=Disabled  DerivativeFilterVariant=ContFilter  NVariant=InternalParameters  NCopyVariant=Disabled  FilterICVariant=InternalICsFilter  IntegratorICVariant=InternalICs  ExternalResetVariant=Disabled  TRSumVariant=Passthrough  SumFdbkVariant=Disabled  SumVariant=Sum_PID  TsampFilterVariant=InternalTs  TsampNgainVariant=Passthrough  TsampIntegralVariant=Passthrough  ExternalSaturationOutDataTypeStr=Inherit: Same as second input
  Sum1 : Sum  Inputs=-+|
  cv [-] : Outport
  wires:
  T_fc [K]/1 -> Sum1/1
  Gain/1 -> PID Controller1/1
  Sum1/1 -> Gain/1
  PID Controller1/1 -> cv [-]/1
  T_fc_ref [K]/1 -> Sum1/2

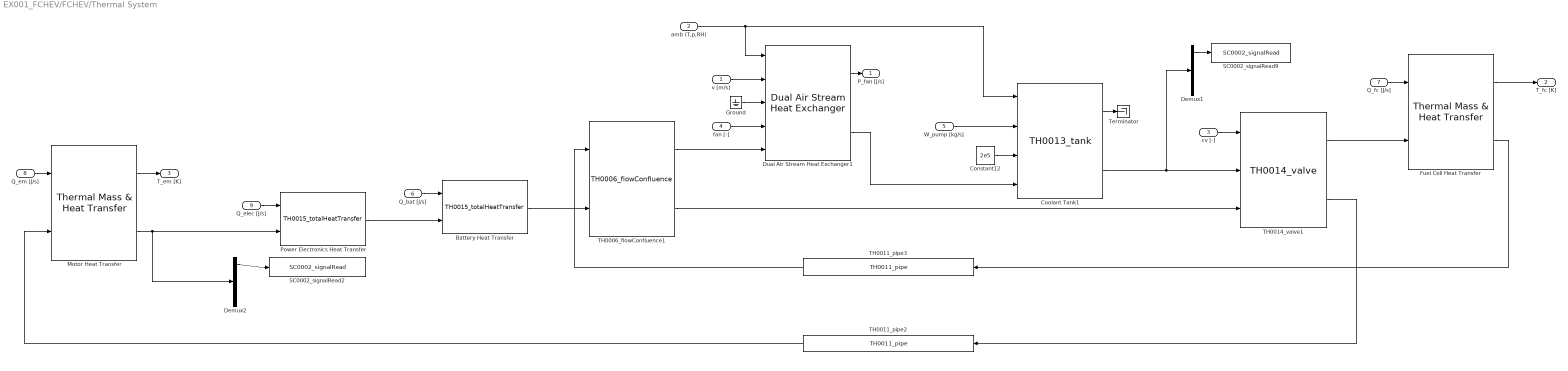
== system EX001_FCHEV/FCHEV/Thermal System ==
  v [m/s] : Inport
  amb (T,p,RH) : Inport  Port=2
  cv [-] : Inport  Port=3
  fan [-] : Inport  Port=4
  W_pump [kg/s] : Inport  Port=5
  Q_bat [J/s] : Inport  Port=6
  Q_fc [J/s] : Inport  Port=7
  Q_em [J/s] : Inport  Port=8
  Q_elec [J/s] : Inport  Port=9
  Battery Heat Transfer : component_lib/Thermal Systems/TH0015_totalHeatTransfer  SystemSampleTime=-1  VariantActivationTime=update diagram  Latency=0  AutoFrameSizeCalculation=off
  Constant12 : Constant  Value=2e5
  Coolant Tank1 : component_lib/Thermal Systems/TH0013_tank  V=5e-3
  Demux1 : Demux  Outputs=3
  Demux2 : Demux  Outputs=3
  Dual Air Stream Heat Exchanger1 : component_lib/Dual Air Stream Heat Exchanger  HtH=1.1  StS=0.95
  Fuel Cell Heat Transfer : component_lib/Thermal Mass & Heat Transfer  n=450*2*10  d=2e-3  L=50e-2  m=100  cp=420  T_0=273 + 20
  Ground : Ground
  Motor Heat Transfer : component_lib/Thermal Mass & Heat Transfer  n=100*3  d=5e-3  L=30e-2  m=200  cp=420  T_0=273 + 20
  Power Electronics Heat Transfer : component_lib/Thermal Systems/TH0015_totalHeatTransfer  SystemSampleTime=-1  VariantActivationTime=update diagram  Latency=0  AutoFrameSizeCalculation=off
  SC0002_signalRead2 : component_lib/Data & Control/SC0002_signalRead  SigName=powerElectronicsTemperature
  SC0002_signalRead9 : component_lib/Data & Control/SC0002_signalRead  SigName=coolantTemperature
  TH0006_flowConfluence1 : component_lib/Thermal Systems/TH0006_flowConfluence  gain=0.01
  TH0011_pipe2 : component_lib/Thermal Systems/TH0011_pipe  d=3e-2  L=2  T_0=273 + 20  p_0=2e5  W_0=2
  TH0011_pipe3 : component_lib/Thermal Systems/TH0011_pipe  d=3e-2  L=2  T_0=273 + 20  p_0=2e5  W_0=2
  TH0014_valve1 : component_lib/Thermal Systems/TH0014_valve  d=10e-2  dr=5e-2  C_d=0.9
  Terminator : Terminator
  P_fan [J/s] : Outport
  T_fc [K] : Outport  Port=2
  T_em [K] : Outport  Port=3
  wires:
  Demux2/1 -> SC0002_signalRead2/1
  TH0014_valve1/2 -> TH0011_pipe2/1
  Power Electronics Heat Transfer/1 -> Battery Heat Transfer/2
  cv [-]/1 -> TH0014_valve1/1
  TH0006_flowConfluence1/1 -> Dual Air Stream Heat Exchanger1/5
  Coolant Tank1/1 -> Terminator/1
  TH0006_flowConfluence1/2 -> TH0014_valve1/3
  amb (T,p,RH)/1 -> Dual Air Stream Heat Exchanger1/1, Coolant Tank1/1
  Battery Heat Transfer/1 -> TH0006_flowConfluence1/2
  Ground/1 -> Dual Air Stream Heat Exchanger1/3
  fan [-]/1 -> Dual Air Stream Heat Exchanger1/4
  Motor Heat Transfer/2 -> Power Electronics Heat Transfer/2, Demux2/1
  Fuel Cell Heat Transfer/2 -> TH0011_pipe3/1
  TH0014_valve1/1 -> Fuel Cell Heat Transfer/2
  Q_elec [J/s]/1 -> Power Electronics Heat Transfer/1
  v [m/s]/1 -> Dual Air Stream Heat Exchanger1/2
  Constant12/1 -> Coolant Tank1/3
  TH0011_pipe3/1 -> TH0006_flowConfluence1/1
  TH0011_pipe2/1 -> Motor Heat Transfer/2
  Q_fc [J/s]/1 -> Fuel Cell Heat Transfer/1
  Q_em [J/s]/1 -> Motor Heat Transfer/1
  Fuel Cell Heat Transfer/1 -> T_fc [K]/1
  Dual Air Stream Heat Exchanger1/1 -> P_fan [J/s]/1
  Motor Heat Transfer/1 -> T_em [K]/1
  Q_bat [J/s]/1 -> Battery Heat Transfer/1
  W_pump [kg/s]/1 -> Coolant Tank1/2
  Coolant Tank1/2 -> Demux1/1, TH0014_valve1/2
  Demux1/1 -> SC0002_signalRead9/1
  Dual Air Stream Heat Exchanger1/2 -> Coolant Tank1/4
